simulink model "conversionYUV"  (R2025a)
settings: Solver=ode3  StartTime=0  StopTime=TFinal  FixedStep=0.2  RelTol=1e-3  EnableMultiTasking=on
settings Model: Creator=The MathWorks, Inc.  LastModifiedBy=The MathWorks, Inc.
settings SolverCC: AlgebraicLoopSolver=TrustRegion
settings DataIOCC: LimitDataPoints=on  SaveFormat=StructureWithTime  SaveOutput=off  SaveTime=off  ReturnWorkspaceOutputs=off
settings OptimizationCC: BlockReduction=off  DefaultParameterBehavior=Inlined  BufferReuse=off  PassReuseOutputArgsThreshold=0.0
settings DebuggingCC: AlgebraicLoopMsg=none  ParameterPrecisionLossMsg=none  ParameterTunabilityLossMsg=error  BusObjectLabelMismatch=error  SFUnexpectedBacktrackingDiag=warning  SFNoUnconditionalDefaultTransitionDiag=warning  SFExecutionAtInitializationDiag=none  ArithmeticOperatorsInVariantConditions=warning
settings HardwareCC: ProdBitPerPointer=32.0  ProdBitPerSizeT=32.0  ProdBitPerPtrDiffT=32.0  ProdLargestAtomicInteger=Long  ProdWordSize=32.0  ProdHWDeviceType=ARM Compatible->ARM 9
settings ModelReferenceCC: EnableRefExpFcnMdlSchedulingChecks=on  PropagateSignalLabelsOutOfModel=off
settings SFSimCC: SimUseLocalCustomCode=off  CustomCodeUndefinedFunction=UseInterfaceOnly
settings RTWCC: GenerateReport=on  RTWUseLocalCustomCode=off  LaunchReport=on  GPUComputeCapability=3.5
settings CodeAppCC: ForceParamTrailComments=on  MaxIdLength=63.0  OperatorAnnotations=on  StateflowObjectComments=on  MATLABSourceComments=on
settings GRTTargetCC: TargetLangStandard=C89/C90 (ANSI)
settings ConfigComp: CovMetricSettings=dw  CovSaveCumulativeToWorkspaceVar=on  CovSaveSingleToWorkspaceVar=on  CovExternalEMLEnable=off  CovSFcnEnable=off

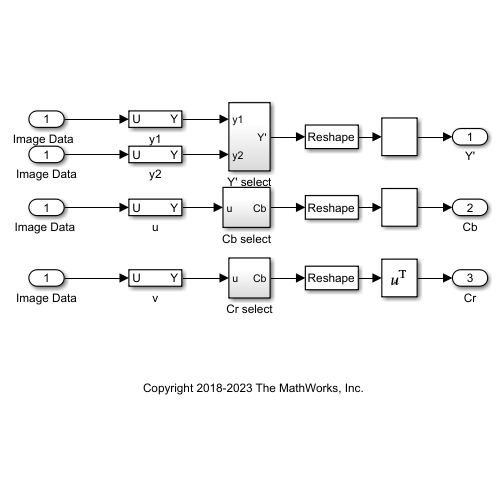
[thumbnail: Simulink's stored preview of the top-level diagram]
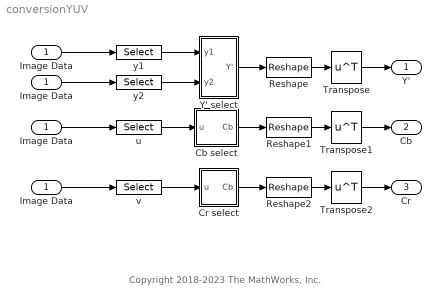
== system conversionYUV ==
  note: Copyright 2018-2023 The MathWorks, Inc.
  Image Data : Inport  OutDataTypeStr=uint8  PortDimensions=[4 9600]  SampleTime=[0.20000000000000001,0]
  " Image Data " : InportShadow  OutDataTypeStr=uint8  PortDimensions=[4 9600]  SampleTime=[0.20000000000000001,0]
  Cb select : Subsystem
  Cr select : Subsystem
  "Image Data " : InportShadow  OutDataTypeStr=uint8  PortDimensions=[4 9600]  SampleTime=[0.20000000000000001,0]
  "Image Data  " : InportShadow  OutDataTypeStr=uint8  PortDimensions=[4 9600]  SampleTime=[0.20000000000000001,0]
  Reshape : Reshape  OutputDimensionality=Customize  OutputDimensions=[160 120]
  Reshape1 : Reshape  OutputDimensionality=Customize  OutputDimensions=[160 120]
  Reshape2 : Reshape  OutputDimensionality=Customize  OutputDimensions=[160 120]
  Transpose : Math  Operator=transpose  SignedPower=on
  Transpose1 : Math  Operator=transpose  SignedPower=on
  Transpose2 : Math  Operator=transpose  SignedPower=on
  Y' select : Subsystem
  u : Selector  NumberOfDimensions=2  InputPortWidth=3  IndexOptions=Index vector (dialog),Select all  Indices=2,1  OutputSizes=1,1
  v : Selector  NumberOfDimensions=2  InputPortWidth=3  IndexOptions=Index vector (dialog),Select all  Indices=4,1  OutputSizes=1,1
  y1 : Selector  NumberOfDimensions=2  InputPortWidth=3  IndexOptions=Index vector (dialog),Select all  Indices=1,1  OutputSizes=1,1
  y2 : Selector  NumberOfDimensions=2  InputPortWidth=3  IndexOptions=Index vector (dialog),Select all  Indices=3,1  OutputSizes=1,1
  Y' : Outport  OutDataTypeStr=uint8  PortDimensions=[120 160]  VectorParamsAs1DForOutWhenUnconnected=off
  Cb : Outport  Port=2  OutDataTypeStr=uint8  PortDimensions=[120 160]  VectorParamsAs1DForOutWhenUnconnected=off
  Cr : Outport  Port=3  OutDataTypeStr=uint8  PortDimensions=[120 160]  VectorParamsAs1DForOutWhenUnconnected=off
  wires:
  Transpose2/1 -> Cr/1
  y1/1 -> Y' select/1(y1)
  Reshape2/1 -> Transpose2/1
  Y' select/1(Y') -> Reshape/1
  Cr select/1(Cb) -> Reshape2/1
  y2/1 -> Y' select/2(y2)
  Reshape1/1 -> Transpose1/1
  u/1 -> Cb select/1(u)
  v/1 -> Cr select/1(u)
  Transpose1/1 -> Cb/1
  Cb select/1(Cb) -> Reshape1/1
  Reshape/1 -> Transpose/1
  Transpose/1 -> Y'/1
  "Image Data "/1 -> u/1
  " Image Data "/1 -> v/1
  Image Data/1 -> y2/1
  "Image Data  "/1 -> y1/1

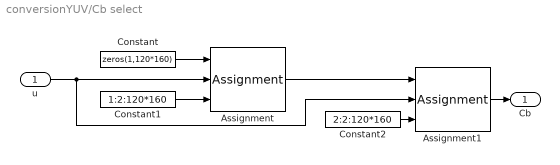
== system conversionYUV/Cb select ==
  u : Inport
  Assignment : Assignment  DiagnosticForDimensions=Warning  IndexOptions=Index vector (port)  Indices=1  OutputSizes=1
  Assignment1 : Assignment  DiagnosticForDimensions=Warning  IndexOptions=Index vector (port)  Indices=1  OutputSizes=1
  Constant : Constant  Value=zeros(1,120*160)  OutDataTypeStr=uint8
  Constant1 : Constant  Value=1:2:120*160
  Constant2 : Constant  Value=2:2:120*160
  Cb : Outport  VectorParamsAs1DForOutWhenUnconnected=off
  wires:
  Constant2/1 -> Assignment1/3
  Constant1/1 -> Assignment/3
  Constant/1 -> Assignment/1
  Assignment1/1 -> Cb/1
  u/1 -> Assignment/2, Assignment1/2
  Assignment/1 -> Assignment1/1

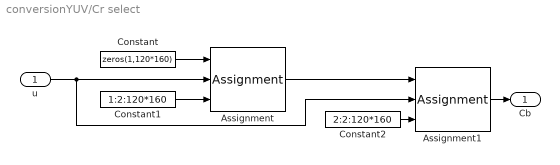
== system conversionYUV/Cr select ==
  u : Inport
  Assignment : Assignment  DiagnosticForDimensions=Warning  IndexOptions=Index vector (port)  Indices=1  OutputSizes=1
  Assignment1 : Assignment  DiagnosticForDimensions=Warning  IndexOptions=Index vector (port)  Indices=1  OutputSizes=1
  Constant : Constant  Value=zeros(1,120*160)  OutDataTypeStr=uint8
  Constant1 : Constant  Value=1:2:120*160
  Constant2 : Constant  Value=2:2:120*160
  Cb : Outport  VectorParamsAs1DForOutWhenUnconnected=off
  wires:
  Assignment/1 -> Assignment1/1
  u/1 -> Assignment1/2, Assignment/2
  Assignment1/1 -> Cb/1
  Constant/1 -> Assignment/1
  Constant1/1 -> Assignment/3
  Constant2/1 -> Assignment1/3

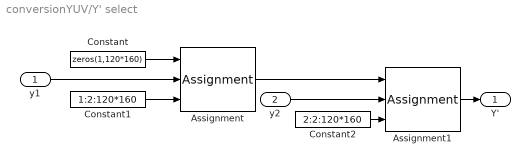
== system conversionYUV/Y' select ==
  y1 : Inport
  y2 : Inport  Port=2
  Assignment : Assignment  DiagnosticForDimensions=Warning  IndexOptions=Index vector (port)  Indices=1  OutputSizes=1
  Assignment1 : Assignment  DiagnosticForDimensions=Warning  IndexOptions=Index vector (port)  Indices=1  OutputSizes=1
  Constant : Constant  Value=zeros(1,120*160)  OutDataTypeStr=uint8
  Constant1 : Constant  Value=1:2:120*160
  Constant2 : Constant  Value=2:2:120*160
  Y' : Outport  VectorParamsAs1DForOutWhenUnconnected=off
  wires:
  y1/1 -> Assignment/2
  Assignment/1 -> Assignment1/1
  y2/1 -> Assignment1/2
  Assignment1/1 -> Y'/1
  Constant/1 -> Assignment/1
  Constant1/1 -> Assignment/3
  Constant2/1 -> Assignment1/3
